simulink model "BatteryModel"  (R2023b)
settings: Solver=VariableStepAuto  StartTime=0.0  StopTime=10.0  RelTol=1e-3
libraries: autolibdatasheetbattery x1
settings Model: Creator=13761  LastModifiedBy=13761

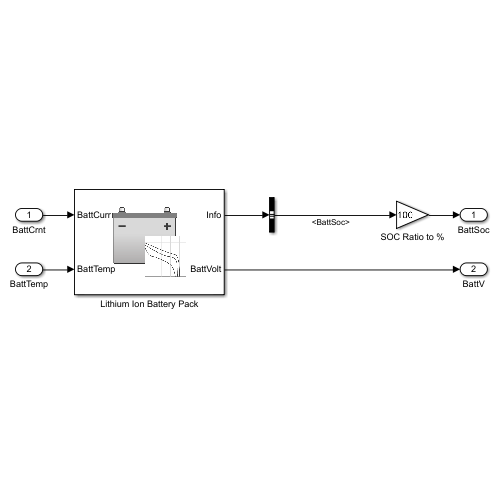
[thumbnail: Simulink's stored preview of the top-level diagram]
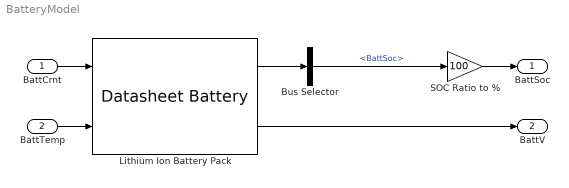
== system BatteryModel ==
  BattCrnt : Inport
  BattTemp : Inport  Port=2
  Bus Selector : BusSelector  OutputSignals=BattSoc
  Lithium Ion Battery Pack : autolibdatasheetbattery/Datasheet Battery  CapacityCtrl=Parameter  OutputVlt=Unfiltered  BattChargeMax=60.8  Em=[2.8 3.228 3.284 3.361 3.408 3.427 3.472 3.477 3.493 3.504 3.516 3.528 3.537 3.545 3.555 3.561 3.566 3.576 3.587 3.589 3.594 3.6 3.608 3.61 3.616 3.619 3.626 3.632 3.637 3.64 3.645 3.646 3.652 3.655 3.658 3.661 3.664 3.668 3.673 3.678 3.68 3.681 3.686 3.692 3.699 3.702 3.705 3.71 3.717 3.723 3.728 3.733 3.735 3.742 3.749 3.755 3.761 3.768 3.773 3.78 3.791 3.798 3.798 3.814 3.818 3.825 3.841 3.846 3.855 3.863 3.877 3.885 3.894 3.907 3.919 3.926 3.935 3.944 3.954 3.964 3.974 3.988 3.998 4.014 4.029 4.034 4.047 4.065 4.074 4.086 4.097 4.131 4.126 4.138 4.15 4.18 4.174 4.187 4.207 4.231 4.221]  CapLUTBp=[0 0.01 0.02 0.03 0.04 0.05 0.06 0.07 0.08 0.09 0.1 0.11 0.12 0.13 0.14 0.15 0.16 0.17 0.18 0.19 0.2 0.21 0.22 0.23 0.24 0.25 0.26 0.27 0.28 0.29 0.3 0.31 0.32 0.33 0.34 0.35 0.36 0.37 0.38 0.39 0.4 0.41 0.42 0.43 0.44 0.45 0.46 0.47 0.48 0.49 0.5 0.51 0.52 0.53 0.54 0.55 0.56 0.57 0.58 0.59 0.6 0.61 0.62 0.63 0.64 0.65 0.66 0.67 0.68 0.69 0.7 0.71 0.72 0.73 0.74 0.75 0.76 0.77 0.78 0.79 0.8 0.81 0.82 0.83 0.84 0.85 0.86 0.87 0.88 0.89 0.9 0.91 0.92 0.93 0.94 0.95 0.96 0.97 0.98 0.99 1]  RInt="[0.004364\t0.004101\t0.00406\t0.003452\t0.003846\t0.004517;0.003639553\t0.003643685\t0.003551349\t0.003225226\t0.003513151\t0.004087354;0.002828222\t0.003115375\t0.003077128\t0.002939098\t0.003187746\t0.00362095;0.002031\t0.002563\t0.002532\t0.00246\t0.002716\t0.003047;0.001443\t0.001825\t0.001795\t0.001778\t0.001924\t0.002234;0.0005603\t0.0007192\t0.0006887\t0.0007557\t0.0007355\t0.001014;0.001028\t0.001338\t0.001\t0.001536\t0.001546\t0.002789]"  BattTempBp=[243.1 253.1 263.1 273.1 283.1 298.1 313.1]  CapSOCBp=[0 0.2 0.4 0.6 0.8 1]  Ns=320/4.2  Np=1  BattCapInit=60.8*0.4  Tc=1/1000  Vinit=4.221  RefBlkName='autolibdatasheetbattery/Datasheet Battery'
  SOC Ratio to % : Gain  Gain=100
  BattSoc : Outport  VectorParamsAs1DForOutWhenUnconnected=off
  BattV : Outport  Port=2  VectorParamsAs1DForOutWhenUnconnected=off
  wires:
  BattTemp/1 -> Lithium Ion Battery Pack/2
  Bus Selector/1 -> SOC Ratio to %/1  "<BattSoc>"
  Lithium Ion Battery Pack/1 -> Bus Selector/1
  SOC Ratio to %/1 -> BattSoc/1
  Lithium Ion Battery Pack/2 -> BattV/1
  BattCrnt/1 -> Lithium Ion Battery Pack/1
